simulink model "plant"  (R2013b)
settings: Solver=ode45  StartTime=0.0  StopTime=10.0  RelTol=1e-3
values from neighbouring files (symbols this model uses):
  w_w = 250    [bla.m]
  w_z = 1.5    [bla.m]
undefined symbols (not defined in the file or in its folder): g, l_p, l_w, m_car, v_R
settings Model: Creator=daniel  LastModifiedBy=daniel

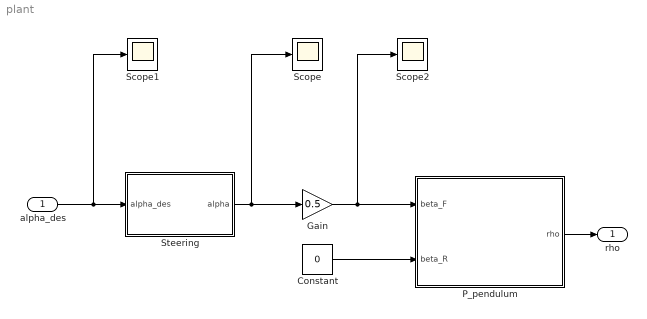
== system plant ==
  alpha_des : Inport
  Constant : Constant  Value=0
  Gain : Gain  Gain=0.5
  P_pendulum : Subsystem
  Scope : Scope
  Scope1 : Scope
      settings: SaveName=ScopeData4
  Scope2 : Scope
      settings: SaveName=ScopeData5
  Steering : Subsystem
  rho : Outport
  wires:
  Constant/1 -> P_pendulum/2(beta_R)
  P_pendulum/1(rho) -> rho/1
  alpha_des/1 -> Scope1/1, Steering/1(alpha_des)
  Steering/1(alpha) -> Scope/1, Gain/1
  Gain/1 -> Scope2/1, P_pendulum/1(beta_F)

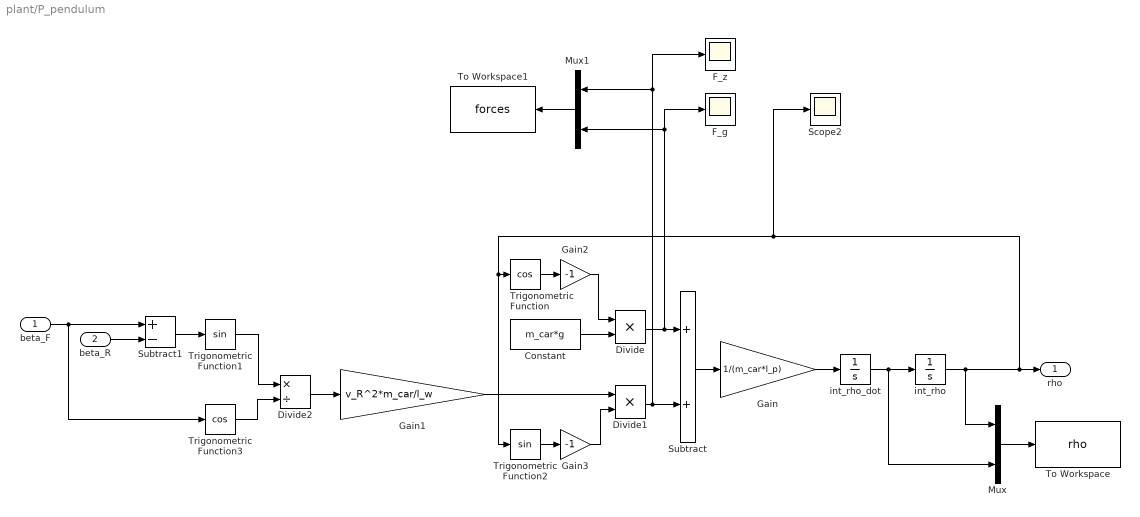
== system plant/P_pendulum ==
  beta_F : Inport
  beta_R : Inport  Port=2
  Constant : Constant  Value=m_car*g
  Divide : Product  Inputs=**
  Divide1 : Product  Inputs=**
  Divide2 : Product  Inputs=*/
  F_g : Scope
      settings: SaveName=ScopeData2
  F_z : Scope
  Gain : Gain  Gain=1/(m_car*l_p)
  Gain1 : Gain  Gain=v_R^2*m_car/l_w
  Gain2 : Gain  Gain=-1
  Gain3 : Gain  Gain=-1
  Mux : Mux  Inputs=2
  Mux1 : Mux  Inputs=2
  Scope2 : Scope
      settings: SaveName=ScopeData3
  Subtract : Sum
  Subtract1 : Sum  Inputs=+-
  To Workspace : ToWorkspace  VariableName=rho  SampleTime=-1  SaveFormat=Timeseries
  To Workspace1 : ToWorkspace  VariableName=forces  SampleTime=-1  SaveFormat=Timeseries
  Trigonometric Function : Trigonometry  Operator=cos
  Trigonometric Function1 : Trigonometry
  Trigonometric Function2 : Trigonometry
  Trigonometric Function3 : Trigonometry  Operator=cos
  int_rho : Integrator  InitialCondition=pi/2+0.01  ContinuousStateAttributes='rho'
  int_rho_dot : Integrator  ContinuousStateAttributes='rho_dot'
  rho : Outport
  wires:
  int_rho_dot/1 -> Mux/2, int_rho/1
  Divide1/1 -> F_z/1, Mux1/1, Subtract/2
  Divide/1 -> F_g/1, Mux1/2, Subtract/1
  beta_F/1 -> Trigonometric Function3/1, Subtract1/1
  beta_R/1 -> Subtract1/2
  Trigonometric Function1/1 -> Divide2/1
  Trigonometric Function/1 -> Gain2/1
  Divide2/1 -> Gain1/1
  Gain/1 -> int_rho_dot/1
  Subtract/1 -> Gain/1
  Subtract1/1 -> Trigonometric Function1/1
  Trigonometric Function2/1 -> Gain3/1
  Mux/1 -> To Workspace/1
  Gain1/1 -> Divide1/1
  Constant/1 -> Divide/2
  Mux1/1 -> To Workspace1/1
  Trigonometric Function3/1 -> Divide2/2
  int_rho/1 -> Scope2/1, Trigonometric Function2/1, Trigonometric Function/1, rho/1, Mux/1
  Gain2/1 -> Divide/1
  Gain3/1 -> Divide1/2

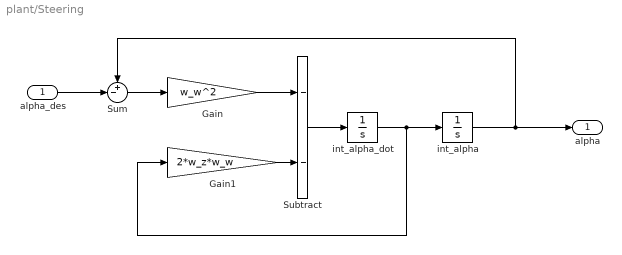
== system plant/Steering ==
  alpha_des : Inport
  Gain : Gain  Gain=w_w^2
  Gain1 : Gain  Gain=2*w_z*w_w
  Subtract : Sum  Inputs=--
  Sum : Sum  Inputs=+-|
  int_alpha : Integrator
  int_alpha_dot : Integrator
  alpha : Outport
  wires:
  int_alpha/1 -> alpha/1, Sum/1
  Subtract/1 -> int_alpha_dot/1
  Sum/1 -> Gain/1
  int_alpha_dot/1 -> Gain1/1, int_alpha/1
  Gain/1 -> Subtract/1
  Gain1/1 -> Subtract/2
  alpha_des/1 -> Sum/2
